simulink model "UKF"  (R2023a)
settings: Solver=VariableStepAuto  StartTime=0.0  StopTime=10.0  RelTol=1e-3
settings Model: Creator=belov  LastModifiedBy=belov

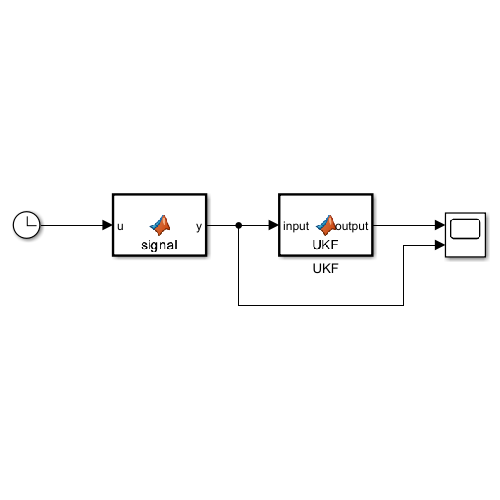
[thumbnail: Simulink's stored preview of the top-level diagram]
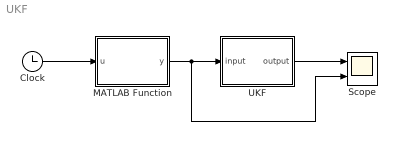
== system UKF ==
  Clock : Clock
  MATLAB Function : MATLAB Function  TreatAsAtomicUnit=on
  Scope : Scope  NumInputPorts=2
  UKF : MATLAB Function  TreatAsAtomicUnit=on
  wires:
  Clock/1 -> MATLAB Function/1(u)
  UKF/1(output) -> Scope/1
  MATLAB Function/1(y) -> Scope/2, UKF/1(input)

== matlab function UKF/UKF ==
  data: input input; output output
function output = UKF(input)

persistent x_last_last P_last_last;
if(isempty(x_last_last))
    x_last_last = 0;
end
if(isempty(P_last_last))
    P_last_last = 1;
end

F = 1;
H = 1;

n = 1;
alpha = 0.2;
kappa = 0;
beta = 2;
lambda = alpha * alpha * (n + kappa) - n;
Q = 0.5;
R = 5;

c = n + lambda;

x_last_lastMatrix = [x_last_last, x_last_last + chol(c * P_last_last)', x_last_last - chol(c * P_last_last)'];
x_last_nowMatrix = F * x_last_lastMatrix;
omegam = [lambda / (n + lambda), lambda / ((n + lambda) * 2), lambda / ((n + lambda) * 2)];
omegac = [lambda / (n + lambda) + (1 - alpha * alpha + beta), lambda / ((n + lambda) * 2), lambda / ((n + lambda) * 2)];

x_last_now = 0;
P_last_now = Q;

for i = 1 : 3
    x_last_now = x_last_now + omegam(i) * x_last_nowMatrix(i);
end
for i = 1 : 3
    P_last_now = P_last_now + omegac(i) * (x_last_nowMatrix(i) - x_last_now) * (x_last_nowMatrix(i) - x_last_now)';
end

x_last_nowMatrix2 = [x_last_now, x_last_now + chol(c * P_last_now)', x_last_now - chol(c * P_last_now)'];
z_last_nowMatrix = H * x_last_nowMatrix2;

z_last_now = 0;

for i = 1 : 3
    z_last_now = z_last_now + omegam(i) * z_last_nowMatrix(i);
end

P_zz = R;
P_xz = 0;

for i = 1 : 3
    P_zz = P_zz + omegac(i) * (z_last_nowMatrix(i) - z_last_now) * (z_last_nowMatrix(i) - z_last_now)';
    P_xz = P_xz + omegac(i) * (x_last_nowMatrix2(i) - x_last_now) * (z_last_nowMatrix(i) - z_last_now)';
end

K_now = P_xz * inv(P_zz);

x_now_now = x_last_now + K_now * (input - z_last_now);
P_now_now = P_last_now - K_now * P_zz * K_now';

x_last_last = x_now_now;
P_last_last = P_now_now;

output = x_now_now;

== matlab function UKF/MATLAB Function ==
  data: u input; y output
function y = signal(u)

y = sin(u);
